simulink model "Simulink_Test_Demo_SC"  (R2025b)
settings: Solver=VariableStepAuto  StartTime=0.0  StopTime=10.0  RelTol=1e-3
settings Model: Creator=P28500  LastModifiedBy=P28500

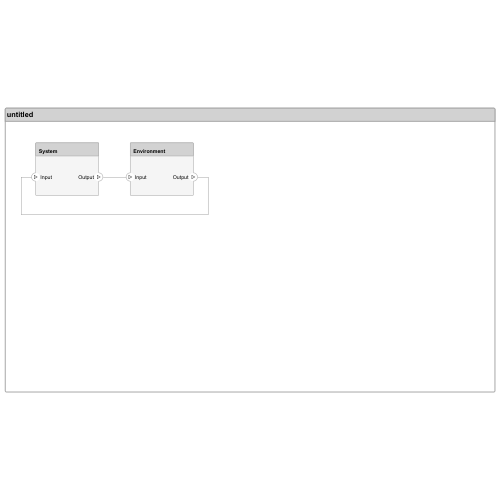
[thumbnail: Simulink's stored preview of the top-level diagram]
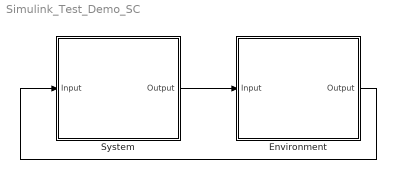
== system Simulink_Test_Demo_SC ==
  Environment : Subsystem
      settings: PortSchema="{\"entries\":[{\"content\":{\"headerSize\":26,\"margin\":15,\"minimumSpacing\":25,\"sides\":[{\"content\":{\"connectorIds\":[\"In1\"]},\"type\":\"ConnectorPlacement.EquallySpacedRectSide\",\"uuid\":\"3a886cb7-c9cf-41d8-94df-ca6edf679de1\"},{\"content\":{\"connectorIds\":[\"Out1\"],\"side\":\"RIGHT\"},\"type\":\"ConnectorPlacement.EquallySpacedRectSide\",\"uuid\":\"2af94dde-4a22-49ae-847c-696d38b17ee1\"},{\"content\":{\"side\":\"TOP\"},\"type\":\"ConnectorPlacement.EquallySpacedRectSide\",\"uuid\":\"bd1c8d54-e67e-4fb8-a84f-0ed45a8dc3b4\"}]},\"type\":\"ConnectorPlacement.EquallySpacedConnector\",\"uuid\":\"2ff7b941-54d0-4c9f-bd5a-d7b41432c1c0\"}],\"packageUris\":[\"http://schema.mathworks.com/mf0/Connector/R2020b\"],\"version\":\"1.0\"}"
  System : Subsystem
      settings: PortSchema="{\"entries\":[{\"content\":{\"headerSize\":26,\"margin\":15,\"minimumSpacing\":25,\"sides\":[{\"content\":{\"connectorIds\":[\"In1\"]},\"type\":\"ConnectorPlacement.EquallySpacedRectSide\",\"uuid\":\"3a886cb7-c9cf-41d8-94df-ca6edf679de1\"},{\"content\":{\"connectorIds\":[\"Out1\"],\"side\":\"RIGHT\"},\"type\":\"ConnectorPlacement.EquallySpacedRectSide\",\"uuid\":\"2af94dde-4a22-49ae-847c-696d38b17ee1\"},{\"content\":{\"side\":\"TOP\"},\"type\":\"ConnectorPlacement.EquallySpacedRectSide\",\"uuid\":\"bd1c8d54-e67e-4fb8-a84f-0ed45a8dc3b4\"}]},\"type\":\"ConnectorPlacement.EquallySpacedConnector\",\"uuid\":\"2ff7b941-54d0-4c9f-bd5a-d7b41432c1c0\"}],\"packageUris\":[\"http://schema.mathworks.com/mf0/Connector/R2020b\"],\"version\":\"1.0\"}"
  wires:
  System/1(Output) -> Environment/1(Input)
  Environment/1(Output) -> System/1(Input)

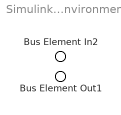
== system Simulink_Test_Demo_SC/Environment ==
  Bus Element In2 : Inport  PortName=Input
  Bus Element Out1 : Outport  PortName=Output

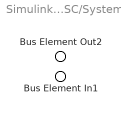
== system Simulink_Test_Demo_SC/System ==
  Bus Element In1 : Inport  PortName=Input
  Bus Element Out2 : Outport  PortName=Output
